simulink model "simulate_QAM"  (R2017a)
settings: Solver=VariableStepAuto  StartTime=0.0  StopTime=.01  RelTol=1e-3
InitFcn:
  | fs = 1e5;
  | frameSize = 1000;
libraries: dspsrcs4 x4, dspfdesign x2
settings Model: Creator=prust  LastModifiedBy=prust

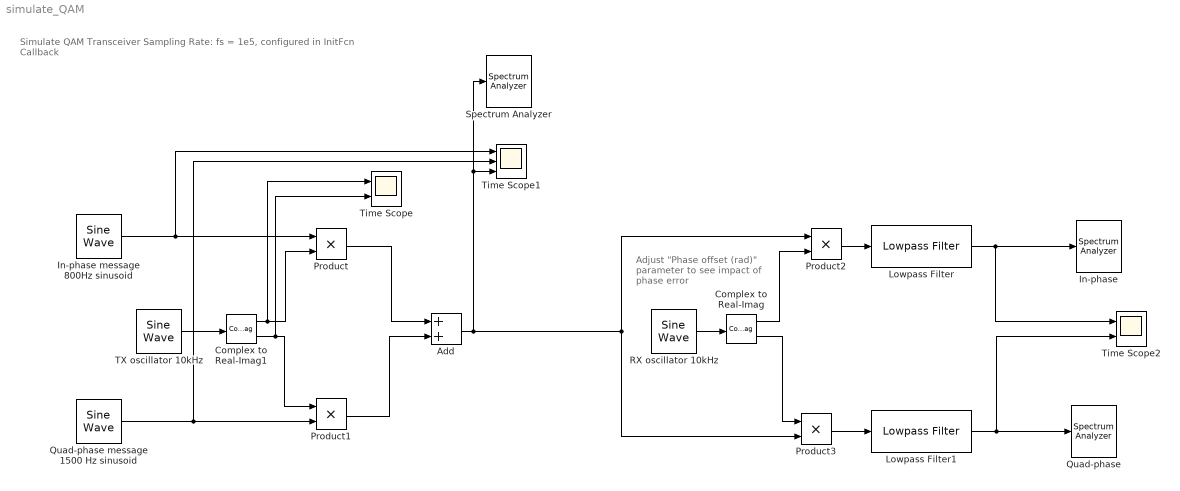
== system simulate_QAM ==
  note: Adjust "Phase offset (rad)" parameter to see impact of phase error
  note: Simulate QAM Transceiver
      | Sampling Rate: fs = 1e5, configured in InitFcn Callback
  Add : Sum
  Complex to Real-Imag : ComplexToRealImag
  Complex to Real-Imag1 : ComplexToRealImag
  In-phase : SpectrumAnalyzer
  In-phase message 800Hz sinusoid : dspsrcs4/Sine Wave  Amplitude=1  Frequency=800  Phase=0  SampleMode=Discrete  OutComplex=Real  CompMethod=Trigonometric fcn  TableSize=Speed  SampleTime=1/fs  SamplesPerFrame=frameSize  ResetState=Restart at time zero  OutputFrames=off  dataType=double  wordLen=16  udDataType=sfix(16)  fracBitsMode=Best precision  numFracBits=15  OutDataTypeStr=double  LastOutDataTypeStr=double
  Lowpass Filter : dspfdesign/Lowpass Filter  FilterType=FIR  DesignForMinimumOrder=off  FilterOrder=40  PassbandFrequency=2e3  StopbandFrequency=2e3  PassbandRipple=0.1  StopbandAttenuation=80  InheritSampleRate=off  SampleRate=fs  SimulateUsing=Interpreted execution  roundingMode=Floor  coeffsDataTypeStr=fixdt(1,16)
  Lowpass Filter1 : dspfdesign/Lowpass Filter  FilterType=FIR  DesignForMinimumOrder=off  FilterOrder=40  PassbandFrequency=2e3  StopbandFrequency=2e3  PassbandRipple=0.1  StopbandAttenuation=80  InheritSampleRate=off  SampleRate=fs  SimulateUsing=Interpreted execution  roundingMode=Floor  coeffsDataTypeStr=fixdt(1,16)
  Product{,1..3} (4 alike) : Product
  Quad-phase : SpectrumAnalyzer
  Quad-phase message 1500 Hz sinusoid : dspsrcs4/Sine Wave  Amplitude=.5  Frequency=1500  Phase=0  SampleMode=Discrete  OutComplex=Real  CompMethod=Trigonometric fcn  TableSize=Speed  SampleTime=1/fs  SamplesPerFrame=frameSize  ResetState=Restart at time zero  OutputFrames=off  dataType=double  wordLen=16  udDataType=sfix(16)  fracBitsMode=Best precision  numFracBits=15  OutDataTypeStr=double  LastOutDataTypeStr=double
  RX oscillator 10kHz : dspsrcs4/Sine Wave  Amplitude=sqrt(2)  Frequency=10000  Phase=0  SampleMode=Discrete  OutComplex=Complex  CompMethod=Trigonometric fcn  TableSize=Speed  SampleTime=1/fs  SamplesPerFrame=frameSize  ResetState=Restart at time zero  OutputFrames=off  dataType=double  wordLen=16  udDataType=sfix(16)  fracBitsMode=Best precision  numFracBits=15  OutDataTypeStr=double  LastOutDataTypeStr=double
  Spectrum Analyzer : SpectrumAnalyzer
  TX oscillator 10kHz : dspsrcs4/Sine Wave  Amplitude=sqrt(2)  Frequency=10000  Phase=0  SampleMode=Discrete  OutComplex=Complex  CompMethod=Trigonometric fcn  TableSize=Speed  SampleTime=1/fs  SamplesPerFrame=frameSize  ResetState=Restart at time zero  OutputFrames=off  dataType=double  wordLen=16  udDataType=sfix(16)  fracBitsMode=Best precision  numFracBits=15  OutDataTypeStr=double  LastOutDataTypeStr=double
  Time Scope : Scope  NumInputPorts=2
  Time Scope1 : Scope  NumInputPorts=3
  Time Scope2 : Scope  NumInputPorts=2
  wires:
  In-phase message 800Hz sinusoid/1 -> Time Scope1/1, Product/1
  Product/1 -> Add/1
  Quad-phase message 1500 Hz sinusoid/1 -> Time Scope1/2, Product1/2
  Product1/1 -> Add/2
  Complex to Real-Imag/1 -> Product2/2
  Add/1 -> Spectrum Analyzer/1, Time Scope1/3, Product3/2, Product2/1
  Product3/1 -> Lowpass Filter1/1
  Product2/1 -> Lowpass Filter/1
  Lowpass Filter/1 -> Time Scope2/1, In-phase/1
  Complex to Real-Imag/2 -> Product3/1
  RX oscillator 10kHz/1 -> Complex to Real-Imag/1
  Lowpass Filter1/1 -> Time Scope2/2, Quad-phase/1
  Complex to Real-Imag1/2 -> Product1/1, Time Scope/2
  TX oscillator 10kHz/1 -> Complex to Real-Imag1/1
  Complex to Real-Imag1/1 -> Product/2, Time Scope/1
